simulink model "observer"  (Simulink 7.7)
settings: Solver=ode45  StartTime=0.0  StopTime=10.0  RelTol=1e-3
values from neighbouring files (symbols this model uses):
  A = load('HW4_Amatrix.dat')    [script1.m]    (also in script2.m; script3.m)
  B = load('HW4_Bmatrix.dat')    [script1.m]    (also in script2.m; script3.m)
  C = load('HW4_Cmatrix.dat')    [script1.m]    (also in script2.m = eye(9); script3.m)
  D = load('HW4_Dmatrix.dat')    [script1.m]    (also in script2.m = zeros(9,3); script3.m = zeros(9,3))
  k = lqr(A,B,Q,R)    [script1.m]    (also in script2.m = LQR(A,B,Q,R); script3.m = LQR(A,B,Q,R))
  L = lqr(A',C',Q1,R1)    [script1.m]
  x0 = [0 0 0 0 0 0 0 0 0]'    [script1.m]    (also in script2.m; script3.m)
settings Model: Creator=Dell  LastModifiedBy=Dell

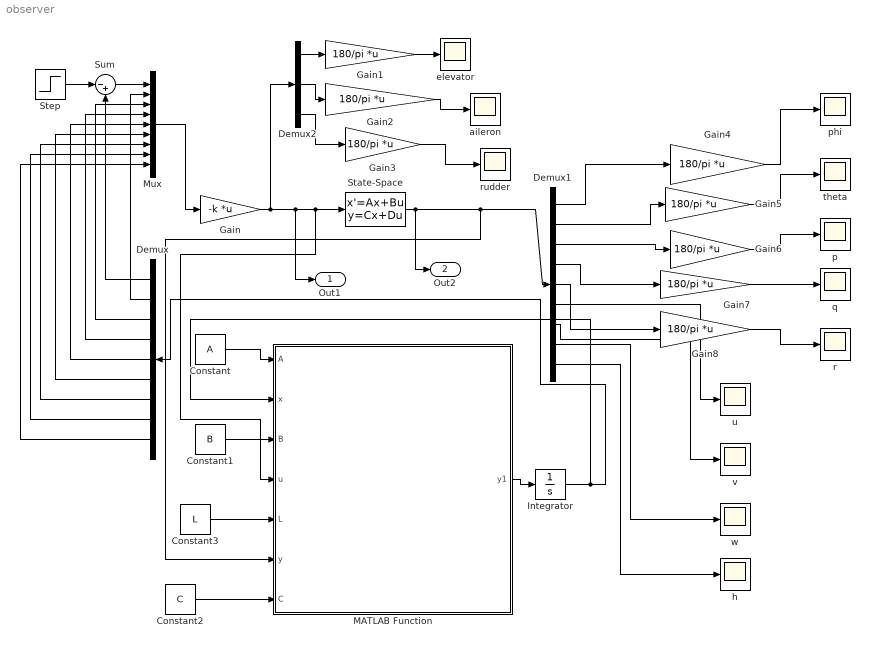
== system observer ==
  Constant : Constant  Value=A
  Constant1 : Constant  Value=B
  Constant2 : Constant  Value=C
  Constant3 : Constant  Value=L
  Demux : Demux  Outputs=9
  Demux1 : Demux  Outputs=9
  Demux2 : Demux  Outputs=3
  Gain : Gain  Gain=-k  Multiplication=Matrix(K*u)
  Gain{1..8} (8 alike) : Gain  Gain=180/pi  Multiplication=Matrix(K*u)
  Integrator : Integrator  InitialCondition=zeros(9,1)
  MATLAB Function : Stateflow chart  TreatAsAtomicUnit=on
  Mux : Mux  Inputs=9
  State-Space : StateSpace  A=A  B=B  C=C  D=D  X0=x0
  Step : Step  Time=0.5  SampleTime=0
  Sum : Sum  Inputs=|-+
  aileron : Scope
      settings: SaveName=ScopeData2
  elevator : Scope
  h : Scope
  p : Scope
      settings: SaveName=ScopeData6
  phi : Scope
      settings: SaveName=ScopeData4
  q : Scope
      settings: SaveName=ScopeData7
  r : Scope
      settings: SaveName=ScopeData8
  rudder : Scope
      settings: SaveName=ScopeData3
  theta : Scope
      settings: SaveName=ScopeData5
  u : Scope
      settings: SaveName=ScopeData9
  v : Scope
      settings: SaveName=ScopeData10
  w : Scope
      settings: SaveName=ScopeData11
  Out1 : Outport
  Out2 : Outport  Port=2
  wires:
  Step/1 -> Sum/1
  Sum/1 -> Mux/1
  Demux/1 -> Sum/2
  Demux/2 -> Mux/2
  Demux/3 -> Mux/3
  Demux/4 -> Mux/4
  Demux/5 -> Mux/5
  Demux/6 -> Mux/6
  Demux/7 -> Mux/7
  Demux/8 -> Mux/8
  Demux/9 -> Mux/9
  Mux/1 -> Gain/1
  Gain/1 -> Demux2/1, Out1/1, State-Space/1, MATLAB Function/4(u)
  Demux2/1 -> Gain1/1
  Demux2/2 -> Gain2/1
  Demux2/3 -> Gain3/1
  Gain1/1 -> elevator/1
  State-Space/1 -> Out2/1, Demux1/1, MATLAB Function/6(y)
  Demux1/1 -> Gain4/1
  Demux1/2 -> Gain5/1
  Demux1/3 -> Gain6/1
  Demux1/4 -> Gain7/1
  Demux1/5 -> Gain8/1
  Demux1/6 -> u/1
  Demux1/7 -> v/1
  Demux1/8 -> w/1
  Demux1/9 -> h/1
  Gain4/1 -> phi/1
  Gain5/1 -> theta/1
  Gain6/1 -> p/1
  Gain7/1 -> q/1
  Gain8/1 -> r/1
  Gain2/1 -> aileron/1
  Gain3/1 -> rudder/1
  MATLAB Function/1(y1) -> Integrator/1
  Integrator/1 -> Demux/1, MATLAB Function/2(x)
  Constant/1 -> MATLAB Function/1(A)
  Constant1/1 -> MATLAB Function/3(B)
  Constant2/1 -> MATLAB Function/7(C)
  Constant3/1 -> MATLAB Function/5(L)

== matlab function MATLAB Function ==
  data: A input double; x input double; B input double; u input double; L input double; y input double; C input double; y1 output double
function y1 = fcn(A,x,B,u,L,y,C)
%#codegen

y1 = A*x + B*u + L*(y-C*x);
